simulink model "ForceReadingSerial"  (R2025b)
settings: Solver=VariableStepAuto  StartTime=0.0  StopTime=inf  RelTol=1e-3
undefined symbols (not defined in the file or in its folder): CR, LF, Ts
libraries: instrumentseriallib x2
settings Model: Creator=mialc  LastModifiedBy=mmm_r

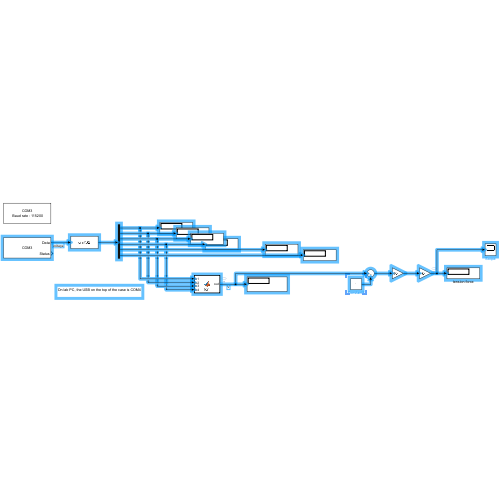
[thumbnail: Simulink's stored preview of the top-level diagram]
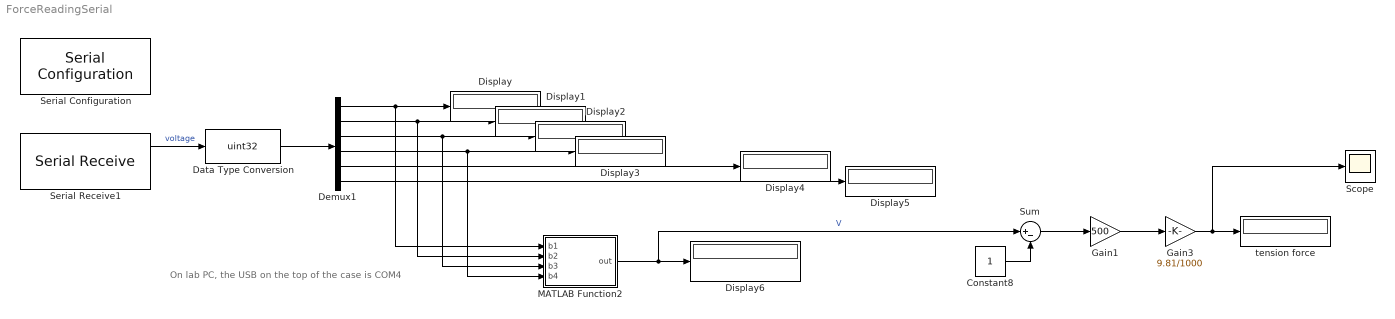
== system ForceReadingSerial ==
  note: On lab PC, the USB on the top of the case is COM4
  Constant8 : Constant
  Data Type Conversion : DataTypeConversion  OutDataTypeStr=uint32  SaturateOnIntegerOverflow=off  RndMeth=Floor
  Demux1 : Demux  Outputs=6
  Display{,1..6} (7 alike) : Display
  Gain1 : Gain  Gain=500
  Gain3 : Gain  Gain=9.81/1000
  MATLAB Function2 : MATLAB Function  TreatAsAtomicUnit=on
  Scope : Scope
      settings: ActiveDisplayYMinimum=-5.8189937737584119  ActiveDisplayYMaximum=3.3209439638257026
  Serial Configuration : instrumentseriallib/Serial Configuration  Priority=-200000  PortSel=COM3  Port=COM3  ComPort=COM3  BaudRate=115200  DataBits=8  Parity=none  StopBits=1  ByteOrder=little-endian  FlowControl=none  Timeout=10  SimulateUsing=Interpreted execution  BlockInModel=on  aMode=1
  Serial Receive1 : instrumentseriallib/Serial Receive  Priority=1  PortSel=COM3  Port=COM3  ComPort=COM3  DataType=uint8  SaveDataType=uint8  ToggleHeader=off  Header=[255]  ToggleDataSize=on  DataSize=[1 6]  ToggleTerminator=off  Terminator=CR/LF ('\r\n')  CustomTerminator=[]  InputFormat=Column major  EnableBlockingMode=off  ActionDataUnavailable=Output last received value  ActionWhenDataUnavailable=Output last received value  CustomValue=0  SampleTime=Ts  SimulateUsing=Interpreted execution  BlockInModel=on  aMode=1  LibraryInUse=instrumentlib
  Sum : Sum  Inputs=|+-
  tension force : Display
  wires:
  Demux1/6 -> Display5/1
  Demux1/3 -> MATLAB Function2/3(b3), Display2/1
  Sum/1 -> Gain1/1
  Demux1/4 -> MATLAB Function2/4(b4), Display3/1
  Demux1/1 -> MATLAB Function2/1(b1), Display/1
  Serial Receive1/1 -> Data Type Conversion/1  "voltage"
  Gain1/1 -> Gain3/1
  Data Type Conversion/1 -> Demux1/1
  Demux1/2 -> MATLAB Function2/2(b2), Display1/1
  Constant8/1 -> Sum/2
  Demux1/5 -> Display4/1
  MATLAB Function2/1(out) -> Display6/1, Sum/1  "V"
  Gain3/1 -> Scope/1, tension force/1

== matlab function ForceReadingSerial/MATLAB Function2 ==
  data: b1 input; out output; b2 input; b3 input; b4 input
function out = fcn(b1, b2, b3, b4)
    raw = uint32(b1) + uint32(b2)*256 + uint32(b3)*256^2 + uint32(b4)*256^3;
    out = double(typecast(raw, 'single'));
end
